simulink model "photovoltaic_cell"  (R2021b)
settings: Solver=VariableStepAuto  StartTime=0.0  StopTime=10.0  RelTol=1e-3
values from neighbouring files (symbols this model uses):
  G = [250; 500; 750; 1000]    [config_simulink.m]    (also in day1.m; day1_try.m)
  I = []    [config_simulink.m]    (also in day1.m = [I_250; I_500; I_750; I_1000]; day1_try.m = [I_250; I_500; I_750; I_1000])
  V = []    [config_simulink.m]    (also in day1.m = [V_250; V_500; V_750; V_1000]; day1_try.m = [V_250; V_500; V_750; V_1000])
settings Model: Creator=tinar  LastModifiedBy=tinar

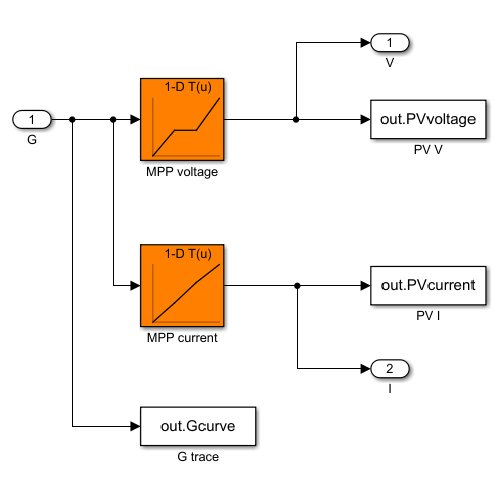
[thumbnail: Simulink's stored preview of the top-level diagram]
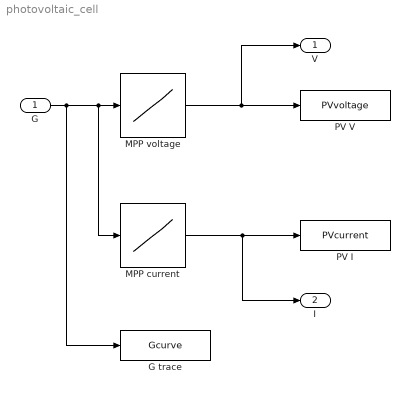
== system photovoltaic_cell ==
  G : Inport
  G trace : ToWorkspace  VariableName=Gcurve  SaveFormat=Timeseries  SampleTime=-1
  MPP current : Lookup_n-D  NumberOfTableDimensions=1  BreakpointsForDimension1=G  Table=I  InternalRulePriority=Speed  RndMeth=Simplest  InputSameDT=on
  MPP voltage : Lookup_n-D  NumberOfTableDimensions=1  BreakpointsForDimension1=G  Table=V  InternalRulePriority=Speed  RndMeth=Simplest  InputSameDT=on
  PV I : ToWorkspace  VariableName=PVcurrent  SaveFormat=Timeseries  SampleTime=-1
  PV V : ToWorkspace  VariableName=PVvoltage  SaveFormat=Timeseries  SampleTime=-1
  V : Outport
  I : Outport  Port=2
  wires:
  MPP voltage/1 -> V/1, PV V/1
  G/1 -> G trace/1, MPP current/1, MPP voltage/1
  MPP current/1 -> I/1, PV I/1
